simulink model "Observador"  (R2014a)
settings: Solver=ode45  StartTime=0.0  StopTime=10  RelTol=1e-3
values from neighbouring files (symbols this model uses):
  A = [ 0 1 ; -1 -3 ]    [Observador1.m]
  A1 = A + 0.3*randn(2,2)    [Observador1.m]
  B = [1 1; 0 1]    [Observador1.m]
  C = [1 0; 0 1]    [Observador1.m]
  D = [ 0 ]    [Observador1.m]
  H = place(A',C',polos)'    [Observador1.m]
settings Model: Creator=unieerisantos  LastModifiedBy=unieerisantos

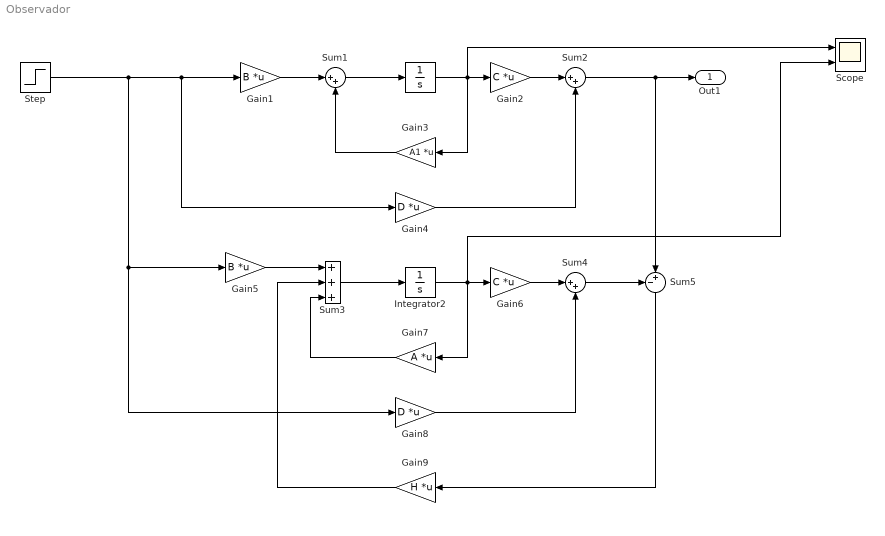
== system Observador ==
  "\t" : Integrator
  Gain1 : Gain  Gain=B  Multiplication=Matrix(K*u)
  Gain2 : Gain  Gain=C  Multiplication=Matrix(K*u)
  Gain3 : Gain  Gain=A1  Multiplication=Matrix(K*u)
  Gain4 : Gain  Gain=D  Multiplication=Matrix(K*u)
  Gain5 : Gain  Gain=B  Multiplication=Matrix(K*u)
  Gain6 : Gain  Gain=C  Multiplication=Matrix(K*u)
  Gain7 : Gain  Gain=A  Multiplication=Matrix(K*u)
  Gain8 : Gain  Gain=D  Multiplication=Matrix(K*u)
  Gain9 : Gain  Gain=H  Multiplication=Matrix(K*u)
  Integrator2 : Integrator
  Scope : Scope  NumInputPorts=2
      settings: YMin=-5~-5  YMax=5~5  SaveName=obs1
  Step : Step  Time=[1 1]  Before=[0 0]  After=[1 1]  SampleTime=0
  Sum1 : Sum  Inputs=|++
  Sum2 : Sum  Inputs=|++
  Sum3 : Sum  Inputs=+++
  Sum4 : Sum  Inputs=|++
  Sum5 : Sum  Inputs=-+|
  Out1 : Outport
  wires:
  Gain1/1 -> Sum1/1
  Sum1/1 -> "\t"/1
  "\t"/1 -> Gain3/1, Gain2/1, Scope/1
  Gain2/1 -> Sum2/1
  Gain3/1 -> Sum1/2
  Gain4/1 -> Sum2/2
  Gain5/1 -> Sum3/1
  Sum3/1 -> Integrator2/1
  Integrator2/1 -> Scope/2, Gain6/1, Gain7/1
  Gain6/1 -> Sum4/1
  Gain8/1 -> Sum4/2
  Gain7/1 -> Sum3/3
  Sum4/1 -> Sum5/1
  Sum5/1 -> Gain9/1
  Gain9/1 -> Sum3/2
  Sum2/1 -> Out1/1, Sum5/2
  Step/1 -> Gain5/1, Gain8/1, Gain4/1, Gain1/1
